simulink model "modelo_covid_aula1"  (R2021b)
settings: Solver=VariableStepAuto  StartTime=0.0  StopTime=1000.0  MaxStep=1  RelTol=1e-3
undefined symbols (not defined in the file): Beta, I0, r, R0, S0
settings Model: Creator=20.01521-6  LastModifiedBy=20.01521-6

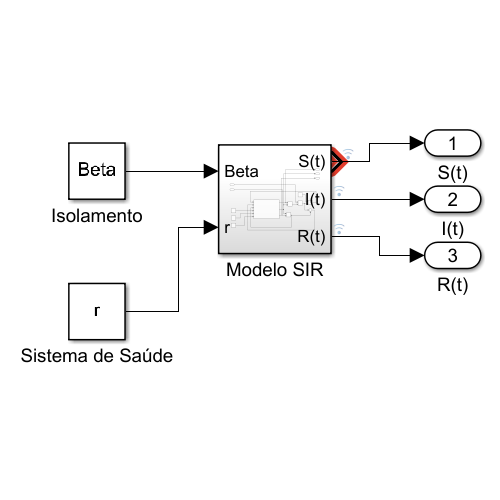
[thumbnail: Simulink's stored preview of the top-level diagram]
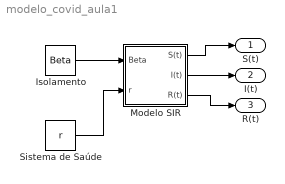
== system modelo_covid_aula1 ==
  Isolamento : Constant  Value=Beta
  Modelo SIR : Subsystem
  Sistema de Saúde : Constant  Value=r
  S(t) : Outport
  I(t) : Outport  Port=2
  R(t) : Outport  Port=3
  wires:
  Isolamento/1 -> Modelo SIR/1(Beta)
  Sistema de Saúde/1 -> Modelo SIR/2(r)
  Modelo SIR/1(S(t)) -> S(t)/1
  Modelo SIR/2(I(t)) -> I(t)/1
  Modelo SIR/3(R(t)) -> R(t)/1

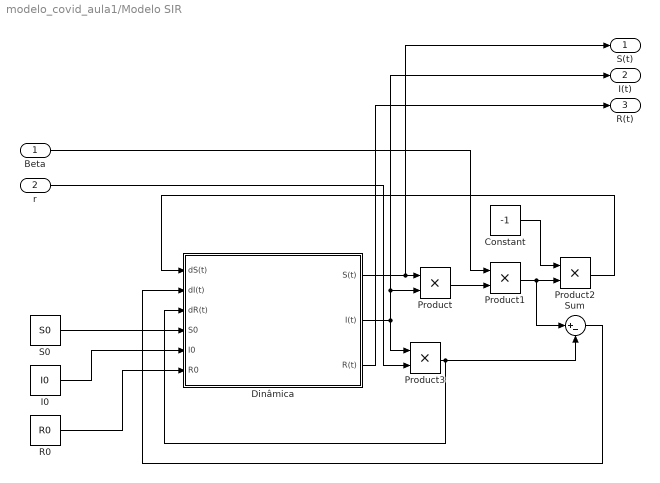
== system modelo_covid_aula1/Modelo SIR ==
  Beta : Inport
  r : Inport  Port=2
  Constant : Constant  Value=-1
  Dinâmica : Subsystem
  I0 : Constant  Value=I0
  Product{,1..3} (4 alike) : Product
  R0 : Constant  Value=R0
  S0 : Constant  Value=S0
  Sum : Sum  Inputs=|+-
  S(t) : Outport
  I(t) : Outport  Port=2
  R(t) : Outport  Port=3
  wires:
  Dinâmica/1(S(t)) -> S(t)/1, Product/1
  Dinâmica/2(I(t)) -> I(t)/1, Product/2, Product3/1
  Product3/1 -> Dinâmica/3(dR(t)), Sum/2
  I0/1 -> Dinâmica/5(I0)
  Product1/1 -> Sum/1, Product2/2
  Dinâmica/3(R(t)) -> R(t)/1
  R0/1 -> Dinâmica/6(R0)
  Beta/1 -> Product1/1
  Product/1 -> Product1/2
  S0/1 -> Dinâmica/4(S0)
  Constant/1 -> Product2/1
  Sum/1 -> Dinâmica/2(dI(t))
  r/1 -> Product3/2
  Product2/1 -> Dinâmica/1(dS(t))

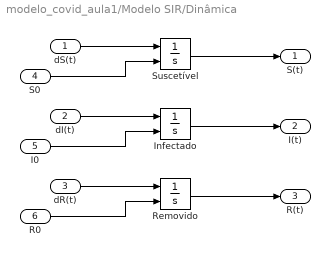
== system modelo_covid_aula1/Modelo SIR/Dinâmica ==
  dS(t) : Inport
  dI(t) : Inport  Port=2
  dR(t) : Inport  Port=3
  S0 : Inport  Port=4
  I0 : Inport  Port=5
  R0 : Inport  Port=6
  Infectado : Integrator  InitialConditionSource=external
  Removido : Integrator  InitialConditionSource=external
  Suscetível : Integrator  InitialConditionSource=external
  S(t) : Outport
  I(t) : Outport  Port=2
  R(t) : Outport  Port=3
  wires:
  Removido/1 -> R(t)/1
  dI(t)/1 -> Infectado/1
  S0/1 -> Suscetível/2
  R0/1 -> Removido/2
  Infectado/1 -> I(t)/1
  I0/1 -> Infectado/2
  Suscetível/1 -> S(t)/1
  dS(t)/1 -> Suscetível/1
  dR(t)/1 -> Removido/1
